simulink model "engine_h_0_2d"  (R2015a)
settings: Solver=ode45  StartTime=0.0  StopTime=250  RelTol=1e-3
settings Model: Creator=Admin  LastModifiedBy=Гена

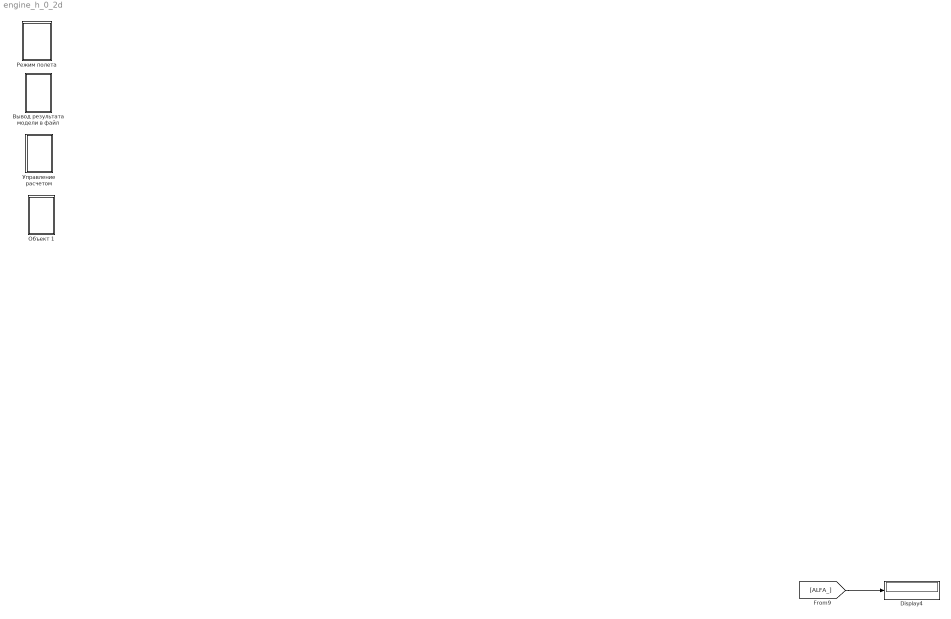
== system engine_h_0_2d ==
  Display4 : Display
  "Вывод результата модели в файл " : Subsystem
  Объект 1 : Subsystem  mask{Iz=2000, Ba=1, S_kr=10}
      mask prompts: Iz "Инерция, относительно оси OZ"; Ba "САХ"; S_kr "Площадь крыла"
  Режим полета : Subsystem  mask(Параметры исходного полета){M_LA=1000, V_0=100, H_0=0.5}
      mask prompts: M_LA "Полетная масса, кг"; V_0 "Скорость полета, м/с"; H_0 "Высота полета, м"
  Управление расчетом : Subsystem  mask{maximum_d_e=30, minimum_d_e=-30, maximum_d_n=30, minimum_d_n=-30, maximum_d_v=30, minimum_d_v=-30, xt_0=1.16}
      mask prompts: maximum_d_e "Максимальное отклонения руля элеронов"; minimum_d_e "Минимальное отклонения руля элеронов"; maximum_d_n "Максимальное отклонения руля направления"; minimum_d_n "Минимальное отклонения руля направления"; maximum_d_v "Максимальное отклонения руля высоты"; minimum_d_v "Минимальное отклонения руля высоты"; xt_0 "Координата центра масс"
  wires:
  [ALFA_] -> Display4/1

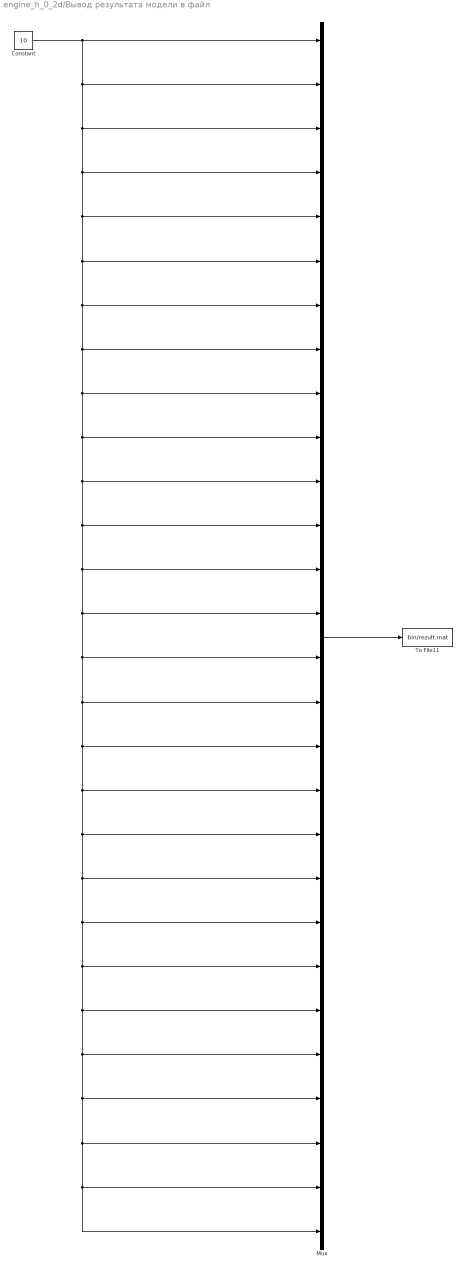
== system engine_h_0_2d/Вывод результата модели в файл  ==
  Constant : Constant  Value=10
  Mux : Mux  Inputs=28
  To File11 : ToFile  Filename=bin/rezult.mat  MatrixName=Variable
  wires:
  Mux/1 -> To File11/1
  Constant/1 -> Mux/11, Mux/28, Mux/27, Mux/26, Mux/25, Mux/24, Mux/23, Mux/22, Mux/21, Mux/20, Mux/19, Mux/18, Mux/17, Mux/16, Mux/15, Mux/14, Mux/13, Mux/12, Mux/10, Mux/9, Mux/8, Mux/7, Mux/6, Mux/5, Mux/4, Mux/3, Mux/2, Mux/1

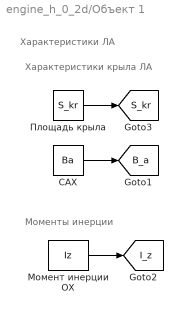
== system engine_h_0_2d/Объект 1 ==
  note: Характеристики ЛА
  note: Моменты инерции
  note: Характеристики крыла ЛА
  Момент инерции ОX : Constant  Value=Iz
  Площадь крыла : Constant  Value=S_kr
  САХ : Constant  Value=Ba
  tag scope: B_a=global, I_z=global, S_kr=global
  wires:
  Площадь крыла/1 -> [S_kr]
  САХ/1 -> [B_a]
  Момент инерции ОX/1 -> [I_z]

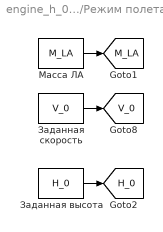
== system engine_h_0_2d/Режим полета ==
  Заданная высота : Constant  Value=H_0
  Заданная скорость : Constant  Value=V_0
  Масса ЛА : Constant  Value=M_LA
  tag scope: H_0=global, M_LA=global, V_0=global
  wires:
  Заданная скорость/1 -> [V_0]
  Масса ЛА/1 -> [M_LA]
  Заданная высота/1 -> [H_0]

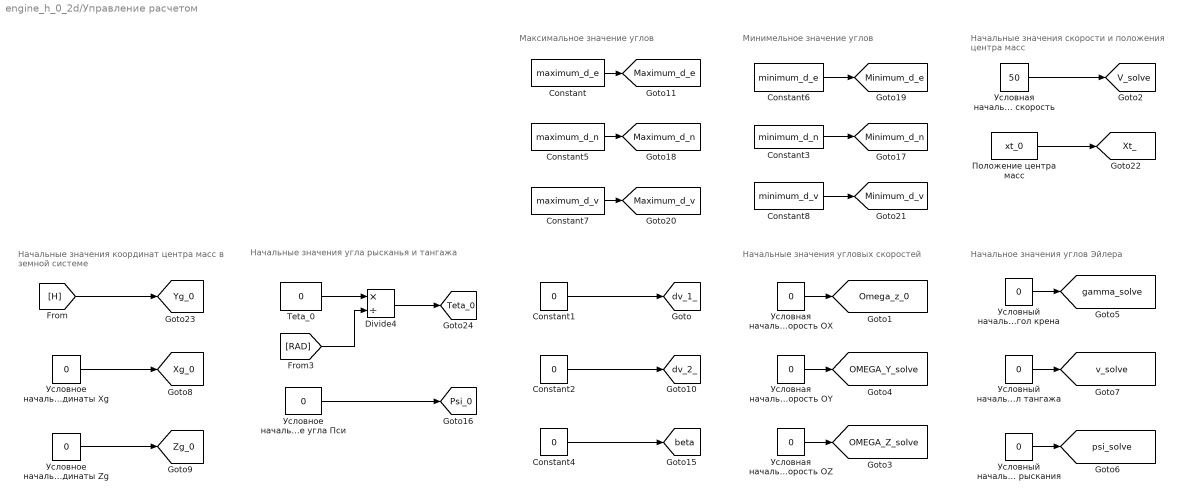
== system engine_h_0_2d/Управление расчетом ==
  note: Начальные значения скорости и
      | положения центра масс
  note: Минимельное значение углов
  note: Максимальное значение углов
  note: Начальное значения углов Эйлера
  note: Начальные значения
      | угловых скоростей
  note: Начальные значения угла рысканья и тангажа
  note: Начальные значения координат
      | центра масс в земной системе
  Constant : Constant  Value=maximum_d_e
  Constant1 : Constant  Value=0
  Constant2 : Constant  Value=0
  Constant3 : Constant  Value=minimum_d_n
  Constant4 : Constant  Value=0
  Constant5 : Constant  Value=maximum_d_n
  Constant6 : Constant  Value=minimum_d_e
  Constant7 : Constant  Value=maximum_d_v
  Constant8 : Constant  Value=minimum_d_v
  Divide4 : Product  Inputs=*/
  Teta_0 : Constant  Value=0
  Положение центра масс : Constant  Value=xt_0
  Условная начальная скорость : Constant  Value=50
  Условная начальная угловая скорость OX : Constant  Value=0
  Условная начальная угловая скорость OY : Constant  Value=0
  Условная начальная угловая скорость OZ : Constant  Value=0
  Условное начальное значение координаты Xg : Constant  Value=0
  Условное начальное значение координаты Zg : Constant  Value=0
  Условное начальное значение угла Пси : Constant  Value=0
  Условный начальный угол крена : Constant  Value=0
  Условный начальный угол рыскания : Constant  Value=0
  Условный начальный угол тангажа : Constant  Value=0
  tag scope: Maximum_d_e=global, Maximum_d_n=global, Maximum_d_v=global, Minimum_d_e=global, Minimum_d_n=global, Minimum_d_v=global, OMEGA_Y_solve=global, OMEGA_Z_solve=global, Omega_z_0=global, Psi_0=global, Teta_0=global, V_solve=global, Xg_0=global, Xt_=global, Yg_0=global, Zg_0=global, beta=global, dv_1_=global, dv_2_=global, gamma_solve=global, psi_solve=global, v_solve=global
  wires:
  Условная начальная скорость/1 -> [V_solve]
  Условная начальная угловая скорость OX/1 -> [Omega_z_0]
  Условная начальная угловая скорость OZ/1 -> [OMEGA_Z_solve]
  Условная начальная угловая скорость OY/1 -> [OMEGA_Y_solve]
  Условный начальный угол крена/1 -> [gamma_solve]
  Условный начальный угол рыскания/1 -> [psi_solve]
  Условный начальный угол тангажа/1 -> [v_solve]
  Constant1/1 -> [dv_1_]
  Constant2/1 -> [dv_2_]
  Constant4/1 -> [beta]
  Условное начальное значение угла Пси/1 -> [Psi_0]
  Constant3/1 -> [Minimum_d_n]
  Constant/1 -> [Maximum_d_e]
  Constant6/1 -> [Minimum_d_e]
  Constant5/1 -> [Maximum_d_n]
  Constant8/1 -> [Minimum_d_v]
  Constant7/1 -> [Maximum_d_v]
  Положение центра масс/1 -> [Xt_]
  Teta_0/1 -> Divide4/1
  [RAD] -> Divide4/2
  Divide4/1 -> [Teta_0]
  Условное начальное значение координаты Xg/1 -> [Xg_0]
  Условное начальное значение координаты Zg/1 -> [Zg_0]
  [H] -> [Yg_0]
